simulink model "sl_groundvehicleDynamics_test"  (R2025b)
settings: Solver=ode45  StartTime=0.0  StopTime=2000  RelTol=1e-5  EnableMultiTasking=on
InitFcn:
  | mdl_robot;
values from neighbouring files (symbols this model uses):
  optimized_waypoints = two_opt_nn_multi_optimisation(waypoints)    [mdl_robot.m]
  scanAngles = linspace(-fov_half,fov_half, 30)    [param.m]
undefined symbols (not defined in the file or in its folder): obstacles, robot
libraries: mobileRoboticsLib x4, simulink x4, simulink_extras x2, sharedTrackingLibrary x1
(part 1 of 2)
settings Model: Creator=sriramn  LastModifiedBy=minhn
settings SolverCC: ZeroCrossAlgorithm=Adaptive  AlgebraicLoopSolver=TrustRegion
settings DataIOCC: LimitDataPoints=on  SaveFormat=Array  ReturnWorkspaceOutputs=off
settings OptimizationCC: ReuseModelBlockBuffer=off  LifeSpan=inf
settings DebuggingCC: SolverPrmCheckMsg=warning  UnconnectedInputMsg=warning  UnconnectedOutputMsg=warning  UnconnectedLineMsg=warning  AllowSymbolicDim=off  SFUnexpectedBacktrackingDiag=warning  SFNoUnconditionalDefaultTransitionDiag=warning  SFExecutionAtInitializationDiag=none  ArithmeticOperatorsInVariantConditions=warning
settings HardwareCC: ProdBitPerPointer=32.0  ProdBitPerSizeT=32.0  ProdBitPerPtrDiffT=32.0  ProdLargestAtomicFloat=None  ProdIntDivRoundTo=Undefined  ProdEndianess=Unspecified  ProdWordSize=32.0  ProdHWDeviceType=32-bit Generic
settings ModelReferenceCC: EnableRefExpFcnMdlSchedulingChecks=on  ModelReferenceMinAlgLoopOccurrences=on  PropagateSignalLabelsOutOfModel=off
settings SFSimCC: SimUseLocalCustomCode=off  CustomCodeUndefinedFunction=UseInterfaceOnly
settings RTWCC: RTWUseLocalCustomCode=off  GPUComputeCapability=3.5
settings CodeAppCC: StateflowObjectComments=on
settings GRTTargetCC: TargetLangStandard=C89/C90 (ANSI)
settings ConfigComp: CovMetricSettings=dw  CovSaveCumulativeToWorkspaceVar=on  CovSaveSingleToWorkspaceVar=on  CovExternalEMLEnable=off  CovSFcnEnable=off
settings SimscapeCC: SimscapeLogDataHistory=5000  SimscapeLogDecimation=1  SimscapeNormalizeSystem=off
settings ConfigurationSet: Description=SimMechanics 2G
settings ExplorerConfigSet: InternalSimMechanicsExplorerSettings="<ExplorerConfiguration><canonicalview>planar_xy</canonicalview><AnimationSetting><BasePlaybackSpeed>1.0</BasePlaybackSpeed><PlaybackSpeedFactor>1.0</PlaybackSpeedFactor></AnimationSetting><TilePanel><TileInfo><Tiles Columns=\"1\" Count=\"1\" Rows=\"1\"><Column Left=\"2\" Weight=\"1\"/><Column Left=\"1628\"/><Row Top=\"2\" Weight=\"1\"/><Row Top=\"1072\"/><Tile Height=\"1\" Width=\"1\" X=\"0\" Y=\"0\"/></Tiles></TileInfo><SceneInfo><SceneViewer><BGColor><R>0.60000002384185791</R><G>0.60000002384185791</G><B>0.60000002384185791</B></BGColor><Camera><Position><X>0.22951840878551699</X><Y>0.32651610611526627</Y><Z>-0.27215421354393321</Z></Position><Center><X>-0.15775714411666431</X><Y>-0.15462825985839526</Y><Z>0.065702552916005602</Z></Center><Up><X>-0.56030137557930915</X><Y>0.72817587161684794</Y><Z>0.39474329445726858</Z></Up><Left>-0.21481383955700509</Left><Right>0.21481383955700509</Right><Bottom>-0.27569784609469139</Bottom><Top>0.27569784609469139</Top></Camera></SceneViewer></SceneInfo></TilePanel></ExplorerConfiguration>"

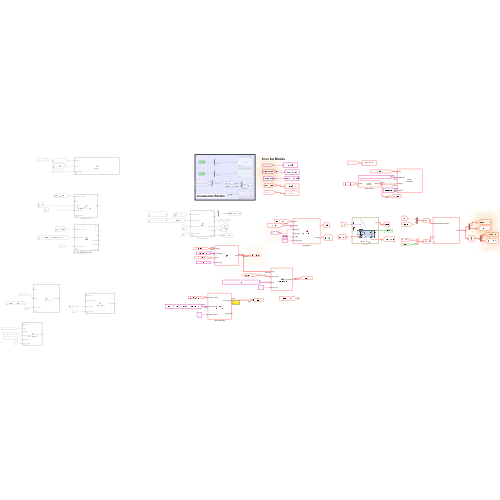
[thumbnail: Simulink's stored preview of the top-level diagram]
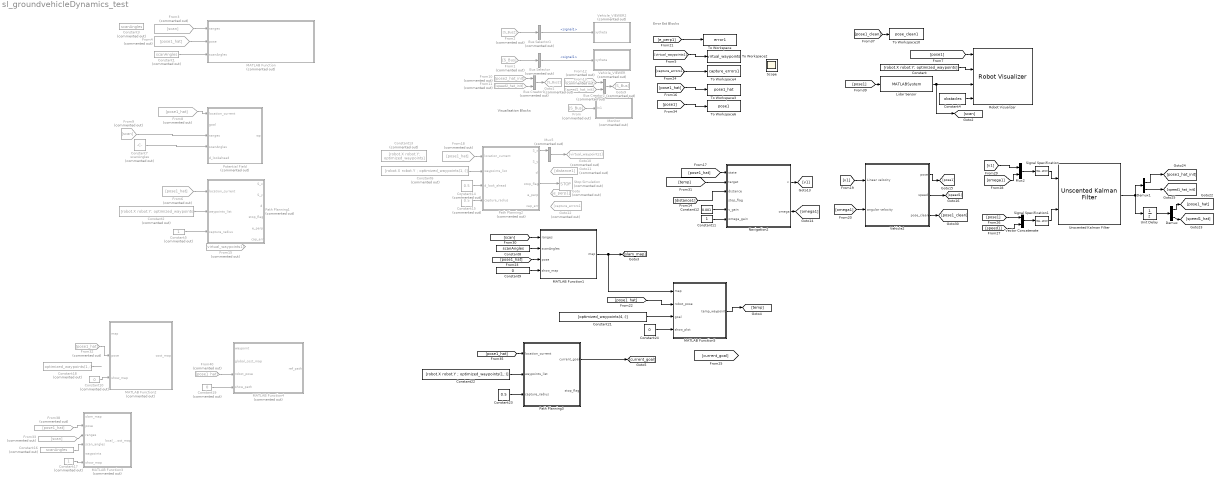
== system sl_groundvehicleDynamics_test ==
  note: Visualisation Blocks
  note: Error Est Blocks
  Bus Creator1 : BusCreator  Commented=on  Inputs=2
  Bus Creator2 : BusCreator  Commented=on  Inputs=2
  Bus Selector : BusSelector  Commented=on  OutputSignals=signal1
  Bus Selector1 : BusSelector  Commented=on  OutputSignals=signal1
  Constant : Constant  Value=[robot.X robot.Y; optimized_waypoints]
  Constant{1,3,7,16} (4 alike) : Constant  Commented=on  Value=scanAngles
  Constant10 : Constant  Commented=on  Value=0
  Constant11 : Constant
  Constant12 : Constant  Value=0.001
  Constant13 : Constant  Commented=on  Value=[robot.X robot.Y; optimized_waypoints]  VectorParams1D=off
  Constant14 : Constant  Commented=on  Value=0.5
  Constant15 : Constant  Commented=on  Value=0.5
  Constant17 : Constant  Commented=on
  Constant18 : Constant  Commented=on  Value=optimized_waypoints(1,:)
  Constant19 : Constant  Commented=on  Value=0
  Constant2 : Constant  Commented=on  Value=[robot.X robot.Y; optimized_waypoints]
  Constant21 : Constant  Value=[optimized_waypoints(4,:)]
  Constant22 : Constant  Value=[robot.X robot.Y ; optimized_waypoints(1,:)]
  Constant23 : Constant  Value=0.5
  Constant24 : Constant  Value=0
  Constant4 : Constant  Value=obstacles
  Constant5 : Constant  Commented=on
  Constant6 : Constant  Commented=on  Value=[robot.X robot.Y ; optimized_waypoints(1,:)]
  Constant8 : Constant  Value=scanAngles
  Constant9 : Constant  Value=0
  Demux : Demux  Outputs=2
  Demux1 : Demux  Outputs=2
  From : From  Commented=on  GotoTag=S_Bus
  From1 : From  Commented=on  GotoTag=S_Bus
  From10 : From  Commented=on  GotoTag=pose2_hat_init
  From11 : From  Commented=on  GotoTag=speed2_hat_init
  From12 : From  Commented=on  GotoTag=pose1_hat_init
  From13 : From  Commented=on  GotoTag=speed1_hat_init
  From15 : From  Commented=on  GotoTag=virtual_waypoints1
  From{4,6,8,18,32,38,40} (7 alike) : From  Commented=on  GotoTag=pose1_hat
  From2 : From  Commented=on  GotoTag=S_Bus2
  From3 : From  Commented=on  GotoTag=scan
  From33 : From  Commented=on  GotoTag=scan
  From9 : From  Commented=on  GotoTag=scan
  Goto : Goto  Commented=on  GotoTag=e_perp1
  Goto1 : Goto  Commented=on  GotoTag=S_Bus2
  Goto10 : Goto  Commented=on  GotoTag=virtual_waypoints1
  Goto11 : Goto  Commented=on  GotoTag=distance1
  Goto12 : Goto  Commented=on  GotoTag=capture_errors1
  Goto9 : Goto  Commented=on  GotoTag=S_Bus
  Lidar Sensor : MATLABSystem  System=LidarSensor  mapName=map  sensorOffset=[ 0, 0 ]  scanAngles=scanAngles  maxRange=30
      mask Type: LidarSensor
  MATLAB Function : MATLAB Function  Commented=on  TreatAsAtomicUnit=on
  MATLAB Function1 : MATLAB Function  TreatAsAtomicUnit=on
  MATLAB Function2 : MATLAB Function  Commented=on  TreatAsAtomicUnit=on
  MATLAB Function3 : MATLAB Function  Commented=on  TreatAsAtomicUnit=on
  MATLAB Function4 : MATLAB Function  Commented=on  TreatAsAtomicUnit=on
  MATLAB Function5 : MATLAB Function  TreatAsAtomicUnit=on
  Monitor : Subsystem  Commented=on
  Mux2 : Mux  Inputs=2
  Mux5 : Mux  Commented=on  Inputs=2
  Navigation2 : MATLAB Function  TreatAsAtomicUnit=on
  Path Planning1 : MATLAB Function  Commented=on  TreatAsAtomicUnit=on
  Path Planning2 : MATLAB Function  Commented=on  TreatAsAtomicUnit=on
  Path Planning3 : MATLAB Function  TreatAsAtomicUnit=on
  Potential Field : MATLAB Function  Commented=on  TreatAsAtomicUnit=on
  Robot Visualizer : mobileRoboticsLib/Environments/Robot Visualizer  robotRadius=0.25  mapName=map  showTrajectory=on  hasWaypoints=on  hasLidar=on  sensorOffset=[ 0, 0 ]  scanAngles=scanAngles  hasObjDetector=on  objDetectorOffset=[ 0, 0 ]  objDetectorAngle=0  objDetectorFOV=pi/4  objDetectorMaxRange=30  objectColors=[ 1, 0, 0; 0, 1, 0; 0, 0, 1 ]  objectMarkers=s
  Signal Specification : SignalSpecification  Dimensions=2
  Signal Specification1 : SignalSpecification  Dimensions=6
  Stop Simulation : Stop  Commented=on
  To Workspace : ToWorkspace  VariableName=error1  SaveFormat=Timeseries  SampleTime=-1
  To Workspace10 : ToWorkspace  VariableName=pose_clean1  SaveFormat=Timeseries  SampleTime=-1
  To Workspace2 : ToWorkspace  VariableName=virtual_waypoints  SaveFormat=Timeseries  SampleTime=-1
  To Workspace3 : ToWorkspace  VariableName=pose1_hat  SaveFormat=Timeseries  SampleTime=-1
  To Workspace4 : ToWorkspace  VariableName=capture_errors1  SaveFormat=Timeseries  SampleTime=-1
  To Workspace6 : ToWorkspace  VariableName=pose1  SaveFormat=Timeseries  SampleTime=-1
  Unit Delay : UnitDelay  InitialCondition=[0;0;0;0;0;0]  SampleTime=-1  HasFrameUpgradeWarning=on
  Unscented Kalman Filter : sharedTrackingLibrary/Unscented Kalman Filter  StateTransitionFcn=fState  HasAdditiveProcessNoise=Additive  ProcessNoise=Q  HasTimeVaryingProcessNoise=off  HasStateTransitionFcnExtraArgument=1  InitialState=initial_state  InitialStateCovariance=P0  Alpha=Alpha  Beta=2  Kappa=0  MeasurementFcn1=hMeas  HasMeasurementEnablePort1=off  HasAdditiveMeasurementNoise1=Additive  MeasurementNoise1=R  HasTimeVaryingMeasurementNoise1=off  HasMeasurementFcnExtraArgument1=0  HasMeasurementWrapping1=on  MeasurementFcn2=myMeasurementFcn  HasMeasurementEnablePort2=off  HasAdditiveMeasurementNoise2=Additive  MeasurementNoise2=1  HasTimeVaryingMeasurementNoise2=off  HasMeasurementFcnExtraArgument2=0  HasMeasurementWrapping2=off  MeasurementFcn3=myMeasurementFcn  HasMeasurementEnablePort3=off  HasAdditiveMeasurementNoise3=Additive  MeasurementNoise3=1  HasTimeVaryingMeasurementNoise3=off  HasMeasurementFcnExtraArgument3=0  HasMeasurementWrapping3=off  MeasurementFcn4=myMeasurementFcn  HasMeasurementEnablePort4=off  HasAdditiveMeasurementNoise4=Additive  MeasurementNoise4=1  HasTimeVaryingMeasurementNoise4=off  HasMeasurementFcnExtraArgument4=0  HasMeasurementWrapping4=off  MeasurementFcn5=myMeasurementFcn  HasMeasurementEnablePort5=off  HasAdditiveMeasurementNoise5=Additive  MeasurementNoise5=1  HasTimeVaryingMeasurementNoise5=off  HasMeasurementFcnExtraArgument5=0  HasMeasurementWrapping5=off  EnableMultirate=off  StateTransitionFcnSampleTime=1  MeasurementFcn1SampleTime=1  MeasurementFcn2SampleTime=1  MeasurementFcn3SampleTime=1  MeasurementFcn4SampleTime=1  MeasurementFcn5SampleTime=1  UseCurrentEstimator=on  OutputStateCovariance=off  DataType=double  SampleTime=0.05  NumberOfMeasurements=1
      settings: LibrarySourceBlock=cstblocks/State Estimation/Unscented Kalman Filter
  Vector Concatenate : Concatenate
  Vehicle2 : Subsystem
      mask Display: image('vehicle.jpg');
  Vehicle_VIEWER : Subsystem  Commented=on  mask{wp_mat=optimized_waypoints, veh_ID_num=1, veh_init_xytheta=[robot.X robot.Y robot.Theta], Ts=0.5}
      mask prompts: wp_mat "Waypoint matrix for arena [x_col, y_col] (m)"; veh_ID_num "Vehicle ID number"; veh_init_xytheta "Initial pose [x,y,theta]"; Ts "Sample time for updating animation (secs)"
      mask TypeOptions veh_ID_num: 1 | 2 | 3 | 4
      mask DialogControl Control2 Prompt: Animate simulation of Differential Drive Robot (DDR)
      mask Display: fprintf('veh_ID=%d',veh_ID_num);
  Vehicle_VIEWER2 : Subsystem  Commented=on  mask{wp_mat=optimized_waypoints, veh_ID_num=2, veh_init_xytheta=[robot.X robot.Y robot.Theta], Ts=0.5}
      mask prompts: wp_mat "Waypoint matrix for arena [x_col, y_col] (m)"; veh_ID_num "Vehicle ID number"; veh_init_xytheta "Initial pose [x,y,theta]"; Ts "Sample time for updating animation (secs)"
      mask TypeOptions veh_ID_num: 1 | 2 | 3 | 4
      mask DialogControl Control2 Prompt: Animate simulation of Differential Drive Robot (DDR)
      mask Display: fprintf('veh_ID=%d',veh_ID_num);
  Scope : Scope
      settings: ActiveDisplayYMinimum=0.07  ActiveDisplayYMaximum=0.09
  wires:
  From12/1 -> Bus Creator2/1
  Bus Creator2/1 -> Goto9/1
  From13/1 -> Bus Creator2/2
  Bus Creator1/1 -> Goto1/1
  From10/1 -> Bus Creator1/1
  From2/1 -> Bus Selector1/1
  From11/1 -> Bus Creator1/2
  From/1 -> Monitor/1(In1)
  Bus Selector1/1 -> Vehicle_VIEWER2/1(xytheta)  "<signal1>"
  Bus Selector/1 -> Vehicle_VIEWER/1(xytheta)  "<signal1>"
  From1/1 -> Bus Selector/1
  Navigation2/2(omega) -> [omega1]
  Vehicle2/1(pose) -> [pose1]
  Constant11/1 -> Navigation2/6(omega_gain)
  [distance1] -> Navigation2/3(distance)
  [v1] -> Vehicle2/1(Linear velocity)
  Constant12/1 -> Navigation2/5(v_gain)
  [omega1] -> Vehicle2/2(angular velocity)
  [pose1_hat] -> Navigation2/1(state)
  Vehicle2/2(speed) -> [speed1]
  Navigation2/1(v) -> [v1]
  [e_perp1] -> To Workspace/1
  [virtual_waypoints1] -> To Workspace2/1
  [pose1_hat] -> To Workspace3/1
  [capture_errors1] -> To Workspace4/1
  Mux2/1 -> Signal Specification/1
  [omega1] -> Mux2/2
  Demux/1 -> [pose1_hat]
  Signal Specification/1 -> Unscented Kalman Filter/1
  Unscented Kalman Filter/1 -> Unit Delay/1, Demux1/1
  Signal Specification1/1 -> Unscented Kalman Filter/2
  [v1] -> Mux2/1
  Demux/2 -> [speed1_hat]
  Unit Delay/1 -> Demux/1
  [pose1] -> Vector Concatenate/1
  Demux1/2 -> [speed1_hat_init]
  Demux1/1 -> [pose1_hat_init]
  [speed1] -> Vector Concatenate/2
  Vector Concatenate/1 -> Signal Specification1/1
  [pose1] -> To Workspace6/1
  [pose1_clean] -> To Workspace10/1
  Vehicle2/3(pose_clean) -> [pose1_clean]
  Constant/1 -> Robot Visualizer/2
  [pose1] -> Robot Visualizer/1
  Constant4/1 -> Robot Visualizer/4
  Lidar Sensor/1 -> [scan], Robot Visualizer/3
  [pose1] -> Lidar Sensor/1
  From3/1 -> MATLAB Function/1(ranges)
  From4/1 -> MATLAB Function/2(pose)
  Constant1/1 -> MATLAB Function/3(scanAngles)
  Constant2/1 -> Path Planning1/2(waypoints_list)
  From6/1 -> Path Planning1/1(location_current)
  Constant5/1 -> Path Planning1/3(capture_radius)
  Mux5/1 -> Goto10/1
  ? -> Goto12/1
  Path Planning2/1(S_x) -> Mux5/1
  Constant14/1 -> Path Planning2/3(d_look_ahead)
  Constant15/1 -> Path Planning2/4(capture_radius)
  ? -> Goto/1
  ? -> Goto11/1
  From18/1 -> Path Planning2/1(location_current)
  ? -> Mux5/2
  From8/1 -> Potential Field/1(location_current)
  From9/1 -> Potential Field/3(ranges)
  Constant7/1 -> Potential Field/4(scanAngles)
  [pose1_hat] -> MATLAB Function1/3(pose)
  Constant8/1 -> MATLAB Function1/2(scanAngles)
  [scan] -> MATLAB Function1/1(ranges)
  [temp] -> Navigation2/2(target)
  Constant9/1 -> MATLAB Function1/4(show_map)
  Path Planning2/4(stop_flag) -> Stop Simulation/1
  From32/1 -> MATLAB Function2/2(pose)
  Constant10/1 -> MATLAB Function2/3(show_map)
  From33/1 -> MATLAB Function3/3(ranges)
  Constant16/1 -> MATLAB Function3/4(scan_angles)
  From38/1 -> MATLAB Function3/2(pose)
  Constant17/1 -> MATLAB Function3/6(show_map)
  Constant6/1 -> Path Planning2/2(waypoints_list)
  From40/1 -> MATLAB Function4/3(robot_pose)
  Constant19/1 -> MATLAB Function4/4(show_path)
  Constant18/1 -> ?
  MATLAB Function1/1(map) -> [slam_map], MATLAB Function5/1(map)
  [pose1_hat] -> MATLAB Function5/2(robot_pose)
  MATLAB Function5/1(temp_waypoint) -> [temp]
  [pose1_hat] -> Path Planning3/1(location_current)
  Constant22/1 -> Path Planning3/2(waypoints_list)
  Constant23/1 -> Path Planning3/3(capture_radius)
  Constant24/1 -> MATLAB Function5/4(show_plot)
  Path Planning3/1(current_goal) -> [current_goal]
  Constant21/1 -> MATLAB Function5/3(goal)

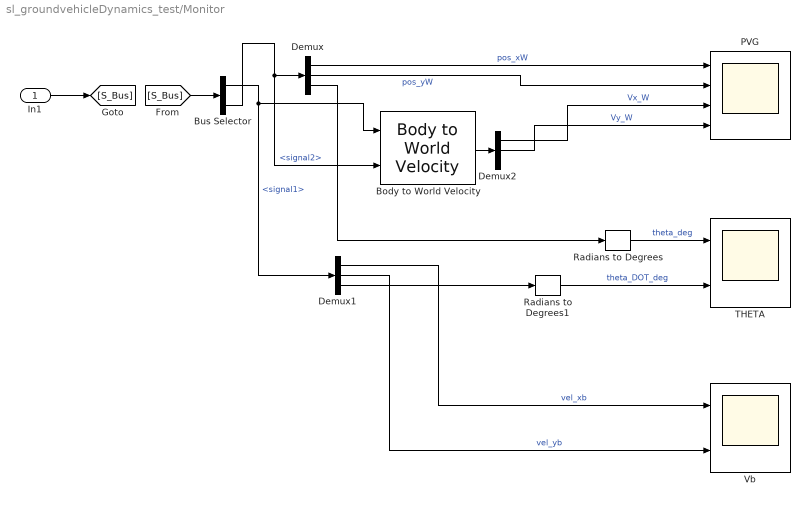
== system sl_groundvehicleDynamics_test/Monitor ==
  In1 : Inport
  Body to World Velocity : mobileRoboticsLib/Utilities/Body to World Velocity
      settings: SourceProductName=Mobile Robotics Simulation Toolbox
  Bus Selector : BusSelector  OutputSignals=signal1,signal2
  Demux : Demux  Outputs=3
  Demux1 : Demux  Outputs=3
  Demux2 : Demux  Outputs=3
  PVG : Scope  NumInputPorts=4
      settings: ActiveDisplayYMinimum=-3.02358  ActiveDisplayYMaximum=27.35477
  Radians to Degrees : simulink_extras/Transformations/Radians to Degrees
  Radians to Degrees1 : simulink_extras/Transformations/Radians to Degrees
  THETA : Scope  NumInputPorts=2
      settings: ActiveDisplayYMinimum=-8.72937  ActiveDisplayYMaximum=60.06611  DataLoggingVariableName=ScopeData2
  Vb : Scope  NumInputPorts=2
      settings: ActiveDisplayYMinimum=0.05577  ActiveDisplayYMaximum=0.8929
  wires:
  In1/1 -> [S_Bus]
  [S_Bus] -> Bus Selector/1
  Demux/1 -> PVG/1  "pos_xW"
  Demux/2 -> PVG/2  "pos_yW"
  Radians to Degrees1/1 -> THETA/2  "theta_DOT_deg"
  Radians to Degrees/1 -> THETA/1  "theta_deg"
  Demux1/3 -> Radians to Degrees1/1
  Demux/3 -> Radians to Degrees/1
  Bus Selector/1 -> Demux1/1, Body to World Velocity/1  "<signal1>"
  Body to World Velocity/1 -> Demux2/1
  Demux2/1 -> PVG/3  "Vx_W"
  Demux2/2 -> PVG/4  "Vy_W"
  Demux1/1 -> Vb/1  "vel_xb"
  Demux1/2 -> Vb/2  "vel_yb"
  Bus Selector/2 -> Body to World Velocity/2, Demux/1  "<signal2>"

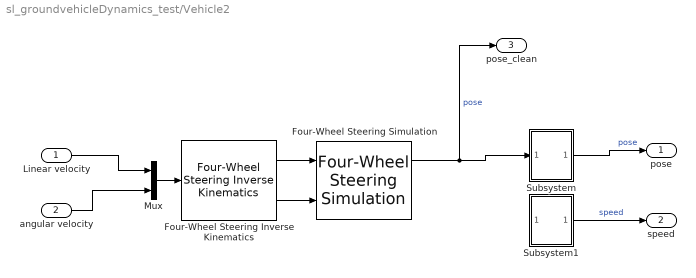
== system sl_groundvehicleDynamics_test/Vehicle2 ==
  Linear velocity : Inport
  angular velocity : Inport  Port=2
  Four-Wheel Steering Inverse Kinematics : mobileRoboticsLib/Kinematic Models/Four-Wheel Steering/Four-Wheel Steering Inverse Kinematics  wheelRadius=0.1  frontWheelDist=0.25  rearWheelDist=0.25  ikMode=Front Steering
      settings: SourceProductName=Mobile Robotics Simulation Toolbox
  Four-Wheel Steering Simulation : mobileRoboticsLib/Kinematic Models/Four-Wheel Steering/Four-Wheel Steering Simulation  wheelRadius=0.1  frontWheelDist=0.25  rearWheelDist=0.25  initX=robot.X  initY=robot.Y  initAngle=robot.Theta  Ts=0.05
      settings: SourceProductName=Mobile Robotics Simulation Toolbox
  Mux : Mux  Inputs=2
  Subsystem : Subsystem
  Subsystem1 : Subsystem
  pose : Outport  VectorParamsAs1DForOutWhenUnconnected=off
  speed : Outport  Port=2
  pose_clean : Outport  Port=3  VectorParamsAs1DForOutWhenUnconnected=off
  wires:
  angular velocity/1 -> Mux/2
  Linear velocity/1 -> Mux/1
  Mux/1 -> Four-Wheel Steering Inverse Kinematics/1
  Four-Wheel Steering Simulation/1 -> pose_clean/1, Subsystem/1(In1)  "pose"
  Four-Wheel Steering Inverse Kinematics/1 -> Four-Wheel Steering Simulation/1
  Four-Wheel Steering Inverse Kinematics/2 -> Four-Wheel Steering Simulation/2
  Subsystem/1(pose) -> pose/1  "pose"
  Subsystem1/1(speed) -> speed/1  "speed"
  ? -> Subsystem1/1(In1)

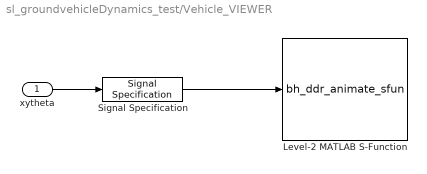
== system sl_groundvehicleDynamics_test/Vehicle_VIEWER ==
  xytheta : Inport
  Level-2 MATLAB S-Function : M-S-Function  FunctionName=bh_ddr_animate_sfun  Parameters=Ts, wp_mat, veh_ID_num, veh_init_xytheta
  Signal Specification : SignalSpecification  Dimensions=3
  wires:
  xytheta/1 -> Signal Specification/1
  Signal Specification/1 -> Level-2 MATLAB S-Function/1

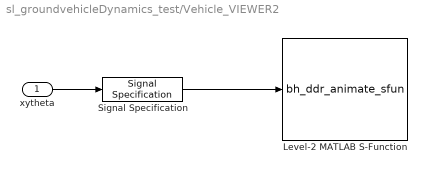
== system sl_groundvehicleDynamics_test/Vehicle_VIEWER2 ==
  xytheta : Inport
  Level-2 MATLAB S-Function : M-S-Function  FunctionName=bh_ddr_animate_sfun  Parameters=Ts, wp_mat, veh_ID_num, veh_init_xytheta
  Signal Specification : SignalSpecification  Dimensions=3
  wires:
  xytheta/1 -> Signal Specification/1
  Signal Specification/1 -> Level-2 MATLAB S-Function/1

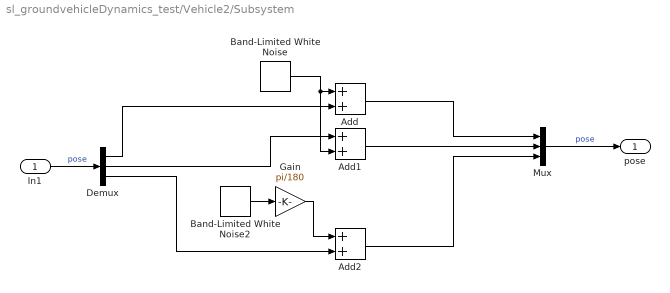
== system sl_groundvehicleDynamics_test/Vehicle2/Subsystem ==
  In1 : Inport
  Add : Sum
  Add1 : Sum
  Add2 : Sum
  Band-Limited White Noise : simulink/Sources/Band-Limited White Noise  Cov=[0.001]  Ts=0.1  seed=[23341]
  Band-Limited White Noise2 : simulink/Sources/Band-Limited White Noise  Cov=[0.41]  Ts=0.1  seed=[23341]
  Demux : Demux  Outputs=3
  Gain : Gain  Gain=pi/180
  Mux : Mux  Inputs=3
  pose : Outport
  wires:
  Add1/1 -> Mux/2
  Add2/1 -> Mux/3
  Demux/2 -> Add1/1
  Band-Limited White Noise2/1 -> Gain/1
  Demux/3 -> Add2/2
  Band-Limited White Noise/1 -> Add1/2, Add/1
  In1/1 -> Demux/1  "pose"
  Demux/1 -> Add/2
  Gain/1 -> Add2/1
  Mux/1 -> pose/1  "pose"
  Add/1 -> Mux/1

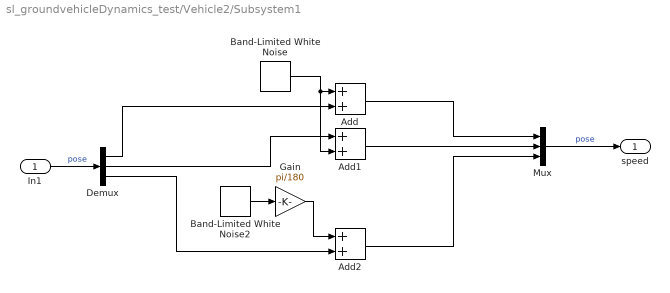
== system sl_groundvehicleDynamics_test/Vehicle2/Subsystem1 ==
  In1 : Inport
  Add : Sum
  Add1 : Sum
  Add2 : Sum
  Band-Limited White Noise : simulink/Sources/Band-Limited White Noise  Cov=[0.001]  Ts=0.1  seed=[23341]
  Band-Limited White Noise2 : simulink/Sources/Band-Limited White Noise  Cov=[0.41]  Ts=0.1  seed=[23341]
  Demux : Demux  Outputs=3
  Gain : Gain  Gain=pi/180
  Mux : Mux  Inputs=3
  speed : Outport
  wires:
  Add1/1 -> Mux/2
  Add2/1 -> Mux/3
  Demux/2 -> Add1/1
  Band-Limited White Noise2/1 -> Gain/1
  Demux/3 -> Add2/2
  Band-Limited White Noise/1 -> Add1/2, Add/1
  In1/1 -> Demux/1  "pose"
  Demux/1 -> Add/2
  Gain/1 -> Add2/1
  Mux/1 -> speed/1  "pose"
  Add/1 -> Mux/1

== matlab function sl_groundvehicleDynamics_test/Path Planning2 ==
  data: location_current input; waypoints_list input; d_look_ahead input; S_x output; S_y output; d output; stop_flag output; capture_radius input; e_perp output; cap_err output
function [S_x, S_y, d, stop_flag, e_perp, cap_err] = RVW(location_current, waypoints_list, d_look_ahead , capture_radius)
% RVWP computes the Rear-View Waypoint (RVWP) for path following
% and cross-track error for plotting
% Modified for Simulink compatibility: returns latest capture error only.

xd = waypoints_list(:,1);
yd = waypoints_list(:,2);

x = location_current(1);
y = location_current(2);

% Persistent variable to remember current waypoint index
persistent n
if isempty(n)
    n = 1;  % Start from the first waypoint
end

stop_flag = 0;
e_perp = 0;      % default
cap_err  = NaN;  % default: no capture at this step

% Distance to next waypoint
if n < length(xd)
    stop_flag = 0;
    d = sqrt((x - xd(n+1))^2 + (y - yd(n+1))^2);

    % Distance & angles for RVWP
    Ru = sqrt((xd(n) - x)^2 + (yd(n) - y)^2);
    theta = atan2(yd(min(n+1,end)) - yd(n), xd(min(n+1,end)) - xd(n));
    theta_u = atan2(y - yd(n), x - xd(n));
    beta = theta - theta_u;
    R = Ru * cos(beta);

    % Compute RVWP
    S_x = xd(n) + (R + d_look_ahead)*cos(theta);
    S_y = yd(n) + (R + d_look_ahead)*sin(theta);

    % Cross-track error (perpendicular to path segment)
    vec_path = [xd(n+1)-xd(n), yd(n+1)-yd(n)];
    vec_to_vehicle = [x - xd(n), y - yd(n)];
    R_path = dot(vec_to_vehicle, vec_path)/norm(vec_path);  % along-track
    e_perp = sqrt(max(0, norm(vec_to_vehicle)^2 - R_path^2)); % perpendicular

    % Waypoint capture check
    if d < capture_radius
        cap_err = d;   % capture error at this waypoint
        n = n + 1;     % Move to next waypoint
    end
else
    % Last waypoint
    d = sqrt((x - xd(n))^2 + (y - yd(n))^2);
    S_x = xd(n);
    S_y = yd(n);
    e_perp = sqrt((x - xd(n))^2 + (y - yd(n))^2);  % distance to final waypoint
    if d < 1
        stop_flag = 1;
        cap_err = d;  % final capture error
    end
end

end

== matlab function sl_groundvehicleDynamics_test/MATLAB Function4 ==
  data: waypoint input; ref_path output; global_cost_map input; robot_pose input; show_path input
function ref_path = planner_server(waypoint, global_cost_map, robot_pose, show_path)
% PLANNER_SERVER - Computes global path to a waypoint using A* for navigation
% Inputs:
%   waypoint         - Target waypoint [x, y, theta] (3x1 double, meters, radians)
%   global_cost_map  - Global costmap (82x104 double, 0=free, 100=obstacle, 1-99=inflation)
%   robot_pose       - Current robot pose [x, y, theta] (3x1 double, meters, radians)
%   show_path        - Boolean flag to visualize path (1x1, set to 0 for codegen)
% Output:
%   ref_path         - Global path [N x 2] double of [x, y] waypoints (N >= 1, max 1000)

% Declare extrinsic functions for visualization (set show_path=0 in Simulink)
coder.extrinsic('imagesc', 'colormap', 'set', 'axis', 'xlabel', 'ylabel', 'title', 'colorbar', 'hold', 'plot');

% Parameters
map_size = [52, 41]; % [m] [x, y]
res = 0.5; % m/cell
rows = 82; % map_size(2)/res
cols = 104; % map_size(1)/res

% Validate inputs
if ~isequal(size(global_cost_map), [rows, cols])
    error('Global costmap must be 82x104');
end
if ~isequal(size(waypoint), [3, 1])
    error('Waypoint must be 3x1');
end
if ~isequal(size(robot_pose), [3, 1])
    error('Robot pose must be 3x1');
end
if ~isscalar(show_path)
    error('show_path must be scalar');
end

% Initialize output as variable-size
ref_path = reshape(robot_pose(1:2), [1 2]); % Default: [1 x 2] at robot_pose
coder.varsize('ref_path', [1000 2], [1 0]); % Min [1 2], max [1000 2]

% Create binary occupancy map for A*
occ_map = binaryOccupancyMap(global_cost_map > 10, res);

% Initialize A* planner
planner = plannerAStarGrid(occ_map);
planner.DiagonalSearch = 'on';
planner.GCost = 'Euclidean';

% Convert poses to grid indices
start = world2grid(robot_pose(1:2), res, map_size);
goal = world2grid(waypoint(1:2), res, map_size);

% Check bounds
if any(start < 1) || start(1) > cols || start(2) > rows || ...
   any(goal < 1) || goal(1) > cols || goal(2) > rows
    warning('Start or goal outside map bounds. Returning robot pose.');
    ref_path = reshape(robot_pose(1:2), [1 2]);
    return;
end

% Plan path
ref_path_grid = plan(planner, start, goal);

% Check planning success
if isempty(ref_path_grid)
    warning('A* planning failed. Returning robot pose.');
    ref_path = reshape(robot_pose(1:2), [1 2]);
    return;
end

% Convert to world coordinates
ref_path = zeros(size(ref_path_grid));
ref_path(:,1) = (ref_path_grid(:,1) - 1) * res; % X
ref_path(:,2) = (ref_path_grid(:,2) - 1) * res; % Y

% Visualization (disabled in Simulink codegen)
if show_path
    imagesc([0, map_size(1)], [0, map_size(2)], global_cost_map);
    colormap(flipud(jet));
    set(gca, 'YDir', 'normal');
    axis equal tight;
    xlabel('X [m]'); ylabel('Y [m]');
    title('Global Costmap with Planned Path');
    colorbar;
    hold on;
    plot(robot_pose(1), robot_pose(2), 'ro', 'MarkerSize', 8, 'LineWidth', 2);
    line_length = 1;
    x_end = robot_pose(1) + line_length * cos(robot_pose(3));
    y_end = robot_pose(2) + line_length * sin(robot_pose(3));
    plot([robot_pose(1), x_end], [robot_pose(2), y_end], 'r-', 'LineWidth', 2);
    plot(waypoint(1), waypoint(2), 'b*', 'MarkerSize', 10);
    plot(ref_path(:,1), ref_path(:,2), 'g-', 'LineWidth', 2);
    hold off;
end

end

% Helper: Convert world coordinates to grid indices
function grid_pos = world2grid(world_pos, res, map_size)
    grid_pos = zeros(1, 2);
    grid_pos(1) = round(world_pos(1)/res) + 1; % X
    grid_pos(2) = round(world_pos(2)/res) + 1; % Y
    grid_pos(1) = max(1, min(grid_pos(1), round(map_size(1)/res)));
    grid_pos(2) = max(1, min(grid_pos(2), round(map_size(2)/res)));
end

== matlab function sl_groundvehicleDynamics_test/MATLAB Function5 ==
  data: map input; temp_waypoint output; robot_pose input; goal input; show_plot input
function temp_waypoint = rrt_navigation(map, robot_pose, goal, show_plot)
% RRT_NAVIGATION - Plans a path using RRT and outputs a temporary waypoint
% Inputs:
%   map        - Binary occupancy grid (82x104, 0=free, 1=occupied)
%   robot_pose - Current robot pose [x, y, theta] (3x1 double, meters, radians)
%   goal       - Goal waypoint [x, y] (2x1 double, meters)
%   show_plot  - Boolean flag to visualize map, tree, and poses (set to 0 for codegen)
% Output:
%   temp_waypoint - Temporary waypoint [x, y] (1x2 double, meters)

% Declare extrinsic functions for visualization (set show_plot=0 in Simulink)
coder.extrinsic('figure', 'imagesc', 'colormap', 'set', 'axis', 'xlabel', 'ylabel', 'title', 'colorbar', 'hold', 'plot', 'clf');

% Parameters
map_size = [52, 41]; % [m] [x, y]
res = 0.5; % m/cell
rows = 82; % map_size(2)/res
cols = 104; % map_size(1)/res
max_iterations = 5000; % Max iterations
step_size = 0.5; % RRT extension step (meters)
goal_bias = 0.1; % Probability to sample goal
goal_radius = 0.5; % Goal reach threshold (meters)
waypoint_dist = 0.5; % Distance to temporary waypoint (meters)

% Validate inputs
if ~isequal(size(map), [rows, cols])
    error('Map must be 82x104');
end
if ~isequal(size(robot_pose), [3, 1])
    error('Robot pose must be 3x1');
end
if ~isequal(size(goal), [2, 1])
    error('Goal must be 2x1');
end
if ~isscalar(show_plot)
    error('show_plot must be scalar');
end

% Initialize output and variables
temp_waypoint = robot_pose(1:2)'; % Default: stay at current position [1x2]
coder.varsize('path', [1000 2], [1 0]);
path = zeros(0, 2); % Initialize as empty
coder.varsize('tree', [10000 3], [1 0]);
tree = zeros(0, 3); % Initialize as empty to ensure definition on all paths

% Check if goal is too close or invalid
if norm(robot_pose(1:2) - goal) < goal_radius
    temp_waypoint = goal'; % Goal reached
    path = [robot_pose(1:2)'; goal'];
else
    % Convert poses to grid coordinates for collision checking
    start_grid = world2grid(robot_pose(1:2), res, map_size);
    goal_grid = world2grid(goal, res, map_size);

    % Check bounds
    if any(start_grid < 1) || start_grid(1) > cols || start_grid(2) > rows || ...
       any(goal_grid < 1) || goal_grid(1) > cols || goal_grid(2) > rows || ...
       map(goal_grid(2), goal_grid(1)) == 1
        warning('Start or goal invalid. Returning robot position.');
        temp_waypoint = robot_pose(1:2)'; % [1x2]
        path = robot_pose(1:2)';
    else
        % Initialize RRT tree: [x, y, parent_index]
        tree = [robot_pose(1:2)', 0]; % Root node at robot_pose, parent=0
        found = false;
        goal_index = 0;

        % RRT loop
        for iter = 1:max_iterations
            % Sample random point
            if rand < goal_bias
                q_rand = goal';
            else
                q_rand = [rand * map_size(1), rand * map_size(2)];
            end

            % Find nearest node in tree
            distances = sqrt(sum((tree(:,1:2) - q_rand).^2, 2));
            [~, nearest_idx] = min(distances);
            q_near = tree(nearest_idx, 1:2);

            % Steer towards q_rand
            direction = q_rand - q_near;
            dist = norm(direction);
            if dist == 0
                continue;
            end
            q_new = q_near + min(step_size, dist) * direction / dist;

            % Check bounds
            q_new_grid = world2grid(q_new, res, map_size);
            if q_new_grid(1) < 1 || q_new_grid(1) > cols || ...
               q_new_grid(2) < 1 || q_new_grid(2) > rows
                continue;
            end

            % Check for collision
            if map(q_new_grid(2), q_new_grid(1)) == 1
                continue;
            end

            % Check if path to q_new is collision-free
            steps = ceil(norm(q_new - q_near) / (res / 2));
            if steps < 2
                steps = 2;
            end
            t = linspace(0, 1, steps);
            collision = false;
            for s = 1:steps
                q_check = q_near + t(s) * (q_new - q_near);
                q_check_grid = world2grid(q_check, res, map_size);
                if q_check_grid(1) < 1 || q_check_grid(1) > cols || ...
                   q_check_grid(2) < 1 || q_check_grid(2) > rows || ...
                   map(q_check_grid(2), q_check_grid(1)) == 1
                    collision = true;
                    break;
                end
            end
            if collision
                continue;
            end

            % Add new node to tree
            tree = [tree; q_new, nearest_idx]; %#ok<AGROW>

            % Check if goal is reached
            if norm(q_new - goal') < goal_radius
                found = true;
                goal_index = size(tree, 1);
                break;
            end
        end

        % Reconstruct path
        if found
            path = goal';
            current_idx = goal_index;
            while current_idx ~= 0
                current_node = tree(current_idx, 1:2);
                path = [current_node; path]; %#ok<AGROW>
                current_idx = tree(current_idx, 3);
            end
            temp_waypoint = select_temp_waypoint(path, robot_pose(1:2)', waypoint_dist);
        else
            warning('RRT failed to reach goal. Returning robot position.');
            path = robot_pose(1:2)';
        end
    end
end

% Visualization
if show_plot
    % Create or switch to figure 2
    figure(4);
    clf; % Clear figure to start fresh
    % Plot map
    imagesc([0, map_size(1)], [0, map_size(2)], map);
    colormap(flipud(gray)); % Black=occupied, white=free
    set(gca, 'YDir', 'normal');
    axis equal tight;
    xlabel('X [m]'); ylabel('Y [m]');
    title('RRT Navigation: Map, Tree, Path, and Poses');
    hold on;

    % Plot RRT tree
    if size(tree, 1) > 1
        for i = 2:size(tree, 1)
            parent_idx = tree(i, 3);
            if parent_idx > 0
                plot([tree(i, 1), tree(parent_idx, 1)], ...
                     [tree(i, 2), tree(parent_idx, 2)], 'c-', 'LineWidth', 0.5); % Tree edges
            end
        end
    end

    % Plot path
    plot(path(:,1), path(:,2), 'r-', 'LineWidth', 2); % Path

    % Plot robot pose
    plot(robot_pose(1), robot_pose(2), 'go', 'MarkerSize', 8, 'LineWidth', 2);
    line_length = 1;
    x_end = robot_pose(1) + line_length * cos(robot_pose(3));
    y_end = robot_pose(2) + line_length * sin(robot_pose(3));
    plot([robot_pose(1), x_end], [robot_pose(2), y_end], 'g-', 'LineWidth', 2);

    % Plot goal
    plot(goal(1), goal(2), 'rx', 'MarkerSize', 10);

    % Plot temporary waypoint
    plot(temp_waypoint(1), temp_waypoint(2), 'm^', 'MarkerSize', 8);

    hold off;
end

end

% Helper: Select temporary waypoint on path
function temp_waypoint = select_temp_waypoint(path, robot_pose, waypoint_dist)
    temp_waypoint = robot_pose; % Default
    for i = 1:size(path, 1)
        dist = norm(path(i, :) - robot_pose);
        if dist > waypoint_dist
            temp_waypoint = path(i, :);
            return;
        end
    end
    % If all points are closer, pick the last one (goal)
    if ~isempty(path)
        temp_waypoint = path(end, :);
    end
end

% Helper: Convert world coordinates to grid indices
function grid_pos = world2grid(world_pos, res, map_size)
    grid_pos = zeros(1, 2);
    grid_pos(1) = round(world_pos(1)/res) + 1; % X
    grid_pos(2) = round(world_pos(2)/res) + 1; % Y
    grid_pos(1) = max(1, min(grid_pos(1), round(map_size(1)/res)));
    grid_pos(2) = max(1, min(grid_pos(2), round(map_size(2)/res)));
end

== matlab function sl_groundvehicleDynamics_test/Path Planning3 ==
  data: location_current input; current_goal output; waypoints_list input; capture_radius input; stop_flag output
function [current_goal, stop_flag] = wp_switch(location_current, waypoints_list, capture_radius)
% WP_SWITCH - Selects the current goal waypoint based on the robot's location
% and a capture radius, for use with path planning (e.g., rrt_navigation).
% Inputs:
%   location_current - Current robot pose [x, y, theta] (3x1 double, meters, radians)
%   waypoints_list   - List of waypoints [x1, y1; x2, y2; ...]' (2xN double, meters)
%   capture_radius    - Radius to switch to next waypoint (scalar double, meters)
% Outputs:
%   current_goal     - Current waypoint to pursue [x, y] (2x1 double, meters)
%   stop_flag        - 1 if all waypoints reached, 0 otherwise (1x1 double)

% Validate inputs


% Extract x, y from waypoints
xd = waypoints_list(:,1); % [1xN]
yd = waypoints_list(:,2); % [1xN]

% Extract current position
x = location_current(1);
y = location_current(2);

% Persistent variable to track current waypoint index
persistent n;
if isempty(n)
    n = 1; % Start from first waypoint
end

% Initialize outputs
current_goal = [xd(n) yd(n)]; % Default: current waypoint [2x1]
stop_flag = 0;

% Check distance to current waypoint
if n <= length(xd)
    d = sqrt((x - xd(n))^2 + (y - yd(n))^2);
    if d < capture_radius
        n = n + 1; % Move to next waypoint
        if n > length(xd)
            stop_flag = 1; % All waypoints reached
            current_goal = [xd(end) yd(end)]; % Stay at last waypoint
        else
            current_goal = [xd(n) yd(n)]; % Next waypoint
        end
    end
else
    stop_flag = 1; % All waypoints reached
    current_goal = [xd(end) yd(end)] % Stay at last waypoint
end

end

== matlab function sl_groundvehicleDynamics_test/Path Planning1 ==
  data: location_current input; S_x output; waypoints_list input; S_y output; d output; stop_flag output; e_perp output; cap_err output; capture_radius input
function [S_x, S_y, d, stop_flag, e_perp, cap_err] = RVW(location_current, waypoints_list, capture_radius)
% RVWP computes the Rear-View Waypoint (RVWP) for path following
% and cross-track error for plotting
% Modified for Simulink compatibility: returns latest capture error only.

xd = waypoints_list(:,1);
yd = waypoints_list(:,2);

x = location_current(1);
y = location_current(2);

% Persistent variable to remember current waypoint index
persistent n
if isempty(n)
    n = 1;  % Start from the first waypoint
end

stop_flag = 0;
e_perp = 0;      % default
cap_err  = NaN;  % default: no capture at this step

% Distance to next waypoint
if n < length(xd)
    stop_flag = 0;
    d = sqrt((x - xd(n+1))^2 + (y - yd(n+1))^2);






    % Waypoint capture check
    if d < capture_radius
        n = n + 1;     % Move to next waypoint
    end
else
    % Last waypoint
    d = sqrt((x - xd(n))^2 + (y - yd(n))^2);
    S_x = xd(n);
    S_y = yd(n);
    e_perp = sqrt((x - xd(n))^2 + (y - yd(n))^2);  % distance to final waypoint
    if d < 1
        stop_flag = 1;
        cap_err = d;  % final capture error
    end
end

end

== matlab function sl_groundvehicleDynamics_test/MATLAB Function ==
  data: ranges input; pose input; scanAngles input
function SLAM_2D(ranges, pose, scanAngles)

persistent first_entry;
persistent xmap;
persistent ymap;
persistent counter;
persistent x_pos;
persistent y_pos;

if isempty(first_entry)
    first_entry = 1;
    xmap    = 0.0;
    ymap    = 0.0;
    counter = 0;
    x_pos   = 0.0;
    y_pos   = 0.0;
end

bearing   = 0;
max_range = 0;
idx       = 1;

xmap  = [xmap; (pose(1) + ranges(:).*cos(pose(3) + scanAngles(:)))];
ymap  = [ymap; (pose(2) + ranges(:).*sin(pose(3) + scanAngles(:)))];

x_pos  = [x_pos; pose(1)];
y_pos  = [y_pos; pose(2)];

if mod(counter,10) == 0
     figure(2),
     plot(xmap,ymap,'r.'); hold on;
     plot(x_pos , y_pos,'b.');
     axis([0 52 0 41])
     xlabel('x pos');ylabel('y pos');
     hold off;
     counter = 0;
end

counter = counter + 1;

== matlab function sl_groundvehicleDynamics_test/Potential Field ==
  data: location_current input; wp output; goal input; ranges input; scanAngles input; d_lookahead input
function wp = Potential_Field_Waypoint(location_current, goal, ranges, scanAngles, d_lookahead)
x = location_current(1);
y = location_current(2);
theta_r = location_current(3);

k_att = 1.0;   % attraction gain
k_rep = 0.1;   % repulsion gain
d0    = 100.0;    % obstacle influence radius

% --- Attractive force ---
F_att = k_att * ([goal(1)-x, goal(2)-y]);

% --- Repulsive force ---
F_rep = [0,0];
obsX = []; obsY = []; repX = []; repY = [];
for i = 1:length(ranges)
    di = ranges(i);
    if di < d0 && di > 0
        % Obstacle position in world frame
        ox = x + di*cos(scanAngles(i) + theta_r);
        oy = y + di*sin(scanAngles(i) + theta_r);

        % Repulsive vector points from obstacle -> robot
        vec_or = [x - ox, y - oy];
        vec_or = vec_or / (norm(vec_or) + eps);  % normalize

        % Magnitude
        Fi = k_rep * (1/di - 1/d0) * (1/di^2) * vec_or;
        F_rep = F_rep + Fi;

        % Store for plotting
        obsX(end+1) = ox;
        obsY(end+1) = oy;
        repX(end+1) = Fi(1);
        repY(end+1) = Fi(2);
    end
end

% --- Total force ---
F_total = F_att + F_rep;
F_total = F_total / (norm(F_total) + eps);

% --- Virtual waypoint ---
wp = [x + d_lookahead*F_total(1), ...
      y + d_lookahead*F_total(2)];

%% --- Plotting live potential field ---
figure(3); clf; hold on; axis equal;
plot(goal(1), goal(2), 'g*', 'MarkerSize', 12, 'LineWidth', 2); % Goal
plot(x, y, 'bo', 'MarkerSize', 8, 'LineWidth', 2);              % Robot
plot(wp(1), wp(2), 'mx', 'MarkerSize', 10, 'LineWidth', 2);     % Virtual waypoint

% Attractive vector (robot → goal)
quiver(x, y, F_att(1), F_att(2), 0, 'g', 'LineWidth', 2, 'MaxHeadSize',2, 'DisplayName','F_{att}');

% Repulsive vectors (from each obstacle)
if ~isempty(obsX)
    quiver(obsX, obsY, repX, repY, 0, 'r', 'LineWidth', 1.5, 'MaxHeadSize',1, 'DisplayName','F_{rep}');
    plot(obsX, obsY, 'ks', 'MarkerSize', 5, 'MarkerFaceColor','k'); % obstacles
end

% Total vector (robot net force)
quiver(x, y, F_total(1), F_total(2), 0, 'b', 'LineWidth', 2, 'MaxHeadSize',2, 'DisplayName','F_{total}');

xlabel('X'); ylabel('Y');
title('Live Potential Field (Robot Frame)');
legend show;
grid on;
drawnow;
end

== matlab function sl_groundvehicleDynamics_test/MATLAB Function1 ==
  data: ranges input; map output; scanAngles input; pose input; show_map input
function map = slam_toolbox(ranges, scanAngles, pose, show_map)
% SLAM-style occupancy grid (debug only, not codegen)
% Inputs:
%   ranges          - lidar ranges (meters)
%   scanAngles      - lidar scan angles (radians)
%   pose- [x, y, theta] in meters, radians
% Output:
%   map             - occupancy grid (2D array, 0=free, 1=occupied)

% Parameters
map_size = [52 41]; % [m] [x, y]
res = 0.5;          % m per cell
cols = round(map_size(1)/res);   % grid cols (x), 104 columns
rows = round(map_size(2)/res);   % grid rows (y), 82 rows
hit_threshold = 0.5;

persistent gridCountsInternal
if isempty(gridCountsInternal)
    gridCountsInternal = zeros(rows, cols);
end

x = pose(1);
y = pose(2);
theta = pose(3);

N = length(ranges);
for i = 1:N
    di = ranges(i);
    if di > 0
        % Relative coordinates
        px_rel = di*cos(scanAngles(i));
        py_rel = di*sin(scanAngles(i));

        % World coordinates (robot pose)
        px = cos(theta)*px_rel - sin(theta)*py_rel + x;
        py = sin(theta)*px_rel + cos(theta)*py_rel + y;

        % Grid index (map origin at (0,0) in bottom-left)
        gx = int32(round(px/res)) + 1; % Shift to 1-based indexing
        gy = int32(round(py/res)) + 1; % Shift to 1-based indexing

        if (gx >= 1) && (gx <= cols) && (gy >= 1) && (gy <= rows)
            gridCountsInternal(gy,gx) = gridCountsInternal(gy,gx) + 1;
        end
    end
end

% Compute and output the thresholded map
map = zeros(rows, cols);
map(gridCountsInternal >= hit_threshold) = 1;
if show_map
    % Plot the map and robot location
    figure(2);
    imagesc([0, 52], [0, 41], map);
    colormap(flipud(gray));
    set(gca, 'YDir', 'normal');
    axis equal tight;
    xlabel('X [m]'); ylabel('Y [m]');
    title('SLAM Occupancy Grid with Robot Location');
    hold on;
    
    % Plot robot's current location
    plot(x, y, 'ro', 'MarkerSize', 8, 'LineWidth', 2); % Red dot for robot position
    
    % Optional: Plot robot orientation as a line (e.g., 1-meter length in direction of theta)
    line_length = 1; % Length of orientation line in meters
    x_end = x + line_length * cos(theta);
    y_end = y + line_length * sin(theta);
    plot([x, x_end], [y, y_end], 'r-', 'LineWidth', 2); % Red line for orientation
    
    hold off;
end
end

== matlab function sl_groundvehicleDynamics_test/MATLAB Function2 ==
  data: map input; cost_map output; pose input; show_map input
function cost_map = global_costmap(map, pose, show_map)
% GLOBAL_COSTMAP - Creates a global costmap from SLAM map for navigation
% Inputs:
%   map      - Binary occupancy grid (82x104, 0=free, 1=occupied) from slam_grid_map
%   pose     - Robot pose [x, y, theta] in meters, radians
%   show_map - Boolean flag to visualize costmap with robot position
% Output:
%   cost_map - Costmap (82x104, 0=free, 100=obstacle, 1-99=inflation)

% Parameters
map_size = [52, 41]; % [m] [x, y]
res = 0.5; % m/cell
rows = round(map_size(2)/res); % 82 rows
cols = round(map_size(1)/res); % 104 cols
inflation_radius = 0.5; % meters, safety buffer around obstacles
max_cost = 100; % Lethal obstacle cost
inflation_decay = 1; % Exponential decay rate for inflation

% Validate inputs
if ~isequal(size(map), [rows, cols])
    error('Input map must be %dx%d', rows, cols);
end
if ~isequal(size(pose), [3, 1]) && ~isequal(size(pose), [1, 3])
    error('Pose must be [x, y, theta]');
end

% Initialize costmap
cost_map = zeros(rows, cols);

% Set lethal obstacles (map=1 -> cost=100)
cost_map(map == 1) = max_cost;

% Apply inflation (buffer around obstacles)
for r = 1:rows
    for c = 1:cols
        if cost_map(r, c) == max_cost
            continue; % Skip obstacles
        end
        % Find distance to nearest obstacle
        min_dist = inf;
        for r2 = 1:rows
            for c2 = 1:cols
                if map(r2, c2) == 1
                    world_dist = res * norm([r-r2, c-c2]); % Distance in meters
                    min_dist = min(min_dist, world_dist);
                end
            end
        end
        % Assign cost based on distance (exponential decay)
        if min_dist <= inflation_radius
            cost_map(r, c) = max_cost * exp(-inflation_decay * min_dist);
        end
    end
end

% Ensure free space is 0
cost_map(map == 0 & cost_map < 1) = 0;

% Visualization
if show_map
    figure(3);
    imagesc([0, map_size(1)], [0, map_size(2)], cost_map);
    colormap(flipud(jet)); % Jet for cost gradient (red=obstacle, blue=free)
    set(gca, 'YDir', 'normal');
    axis equal tight;
    xlabel('X [m]'); ylabel('Y [m]');
    title('Global Costmap with Robot Position');
    colorbar; % Show cost scale
    hold on;
    % Plot robot position
    plot(pose(1), pose(2), 'ro', 'MarkerSize', 8, 'LineWidth', 2);
    % Plot orientation (1m line)
    line_length = 1;
    x_end = pose(1) + line_length * cos(pose(3));
    y_end = pose(2) + line_length * sin(pose(3));
    plot([pose(1), x_end], [pose(2), y_end], 'r-', 'LineWidth', 2);
    hold off;
end

end

== matlab function sl_groundvehicleDynamics_test/Navigation2 ==
  data: state input; v output; omega output; target input; distance input; stop_flag input; v_gain input; omega_gain input
function [v, omega] = pure_pursuit(state, target, distance, stop_flag, v_gain, omega_gain)
%PURE_PURSUIT Compute linear and angular velocity using pure pursuit
%   state: [x, y, theta]
%   target: [x_target, y_target]
%   distance: distance to target
%   stop_flag: 0 = move, 1 = stop



% Linear velocity (minimum 0.5 m/s)
v = distance * v_gain;  % Proportional Control
v = max(v, 1);
%v = 30;
% Relative position
dx = target(1) - state(1);
dy = target(2) - state(2);

% Line-of-sight angle
gamma = atan2(dy, dx);

% Robot orientation
theta = state(3);

% Pure pursuit angular velocity
omega = omega_gain * angdiff(theta, gamma);
if stop_flag == 1
    v = 0;
    omega = 0;
    return;
end
end
